simulink model "Model_Test"  (R2024a)
settings: Solver=FixedStepAuto  StartTime=0.0  StopTime=10000000  FixedStep=0.01  RelTol=1e-3
settings Model: Creator=Djbut  LastModifiedBy=Djbut

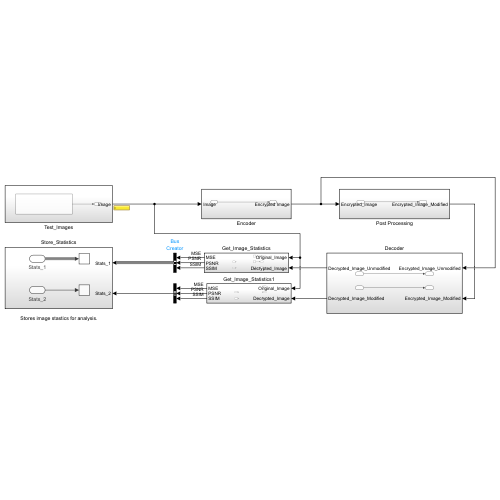
[thumbnail: Simulink's stored preview of the top-level diagram]
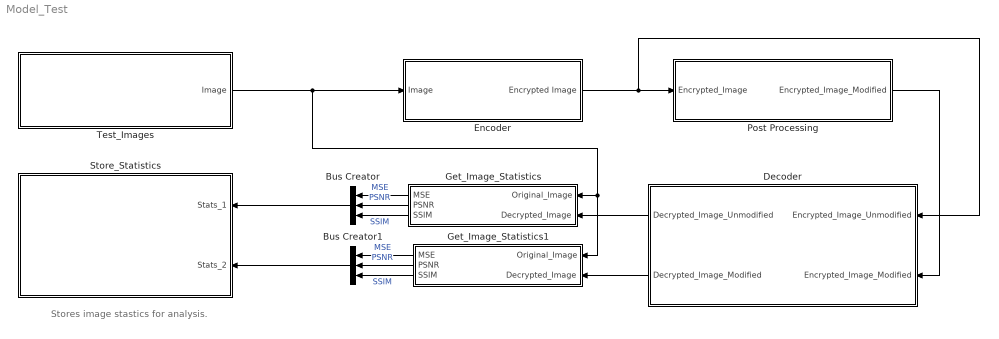
== system Model_Test ==
  note: Stores image stastics for analysis.
  Bus Creator : BusCreator  Inputs=3
  Bus Creator1 : BusCreator  Inputs=3
  Decoder : Subsystem
  Encoder : Subsystem
  Get_Image_Statistics : Subsystem
  Get_Image_Statistics1 : Subsystem
  Post Processing : Subsystem
  Store_Statistics : Subsystem
  Test_Images : Subsystem
  wires:
  Decoder/1(Decrypted_Image_Unmodified) -> Get_Image_Statistics/2(Decrypted_Image)
  Post Processing/1(Encrypted_Image_Modified) -> Decoder/2(Encrypted_Image_Modified)
  Decoder/2(Decrypted_Image_Modified) -> Get_Image_Statistics1/2(Decrypted_Image)
  Encoder/1(Encrypted Image) -> Decoder/1(Encrypted_Image_Unmodified), Post Processing/1(Encrypted_Image)
  Test_Images/1(Image) -> Get_Image_Statistics1/1(Original_Image), Get_Image_Statistics/1(Original_Image), Encoder/1(Image)
  Get_Image_Statistics/1(MSE) -> Bus Creator/1  "MSE"
  Get_Image_Statistics/2(PSNR) -> Bus Creator/2  "PSNR"
  Get_Image_Statistics/3(SSIM) -> Bus Creator/3  "SSIM"
  Bus Creator/1 -> Store_Statistics/1(Stats_1)
  Get_Image_Statistics1/1(MSE) -> Bus Creator1/1  "MSE"
  Get_Image_Statistics1/2(PSNR) -> Bus Creator1/2  "PSNR"
  Get_Image_Statistics1/3(SSIM) -> Bus Creator1/3  "SSIM"
  Bus Creator1/1 -> Store_Statistics/2(Stats_2)

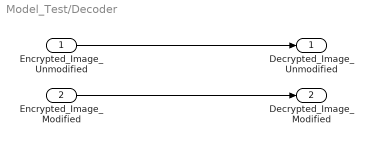
== system Model_Test/Decoder ==
  Encrypted_Image_Unmodified : Inport
  Encrypted_Image_Modified : Inport  Port=2
  Decrypted_Image_Unmodified : Outport
  Decrypted_Image_Modified : Outport  Port=2
  wires:
  Encrypted_Image_Unmodified/1 -> Decrypted_Image_Unmodified/1
  Encrypted_Image_Modified/1 -> Decrypted_Image_Modified/1

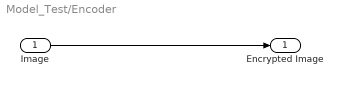
== system Model_Test/Encoder ==
  Image : Inport
  Encrypted Image : Outport
  wires:
  Image/1 -> Encrypted Image/1

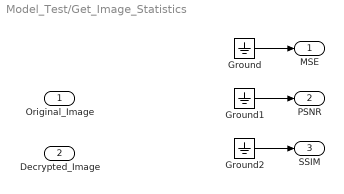
== system Model_Test/Get_Image_Statistics ==
  Original_Image : Inport
  Decrypted_Image : Inport  Port=2
  Ground : Ground
  Ground1 : Ground
  Ground2 : Ground
  MSE : Outport  OutDataTypeStr=int64
  PSNR : Outport  Port=2  OutDataTypeStr=int64
  SSIM : Outport  Port=3  OutDataTypeStr=int64
  wires:
  Ground/1 -> MSE/1
  Ground1/1 -> PSNR/1
  Ground2/1 -> SSIM/1

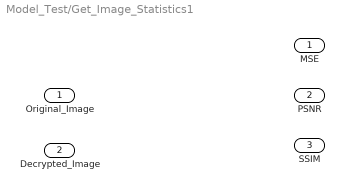
== system Model_Test/Get_Image_Statistics1 ==
  Original_Image : Inport
  Decrypted_Image : Inport  Port=2
  MSE : Outport
  PSNR : Outport  Port=2
  SSIM : Outport  Port=3

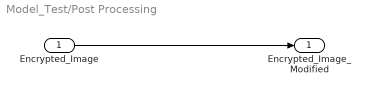
== system Model_Test/Post Processing ==
  Encrypted_Image : Inport
  Encrypted_Image_Modified : Outport
  wires:
  Encrypted_Image/1 -> Encrypted_Image_Modified/1

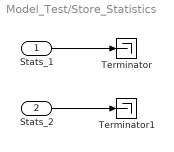
== system Model_Test/Store_Statistics ==
  Stats_1 : Inport
  Stats_2 : Inport  Port=2
  Terminator : Terminator
  Terminator1 : Terminator
  wires:
  Stats_1/1 -> Terminator/1
  Stats_2/1 -> Terminator1/1

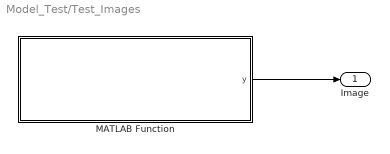
== system Model_Test/Test_Images ==
  MATLAB Function : MATLAB Function  TreatAsAtomicUnit=on
  Image : Outport
  wires:
  MATLAB Function/1(y) -> Image/1

== matlab function Model_Test/Test_Images/MATLAB Function ==
  data: y output
function y = get_images()

y = 0;
